simulink model "dynamic_vibration_absorb"  (R2020a)
settings: Solver=VariableStepAuto  StartTime=0.0  StopTime=50  RelTol=1e-3
PostLoadFcn:
  | m1=1/100
  | b=50
  | k1=50
  | m2=1/2
  | k2=0.9
settings Model: Creator=I3  LastModifiedBy=I3

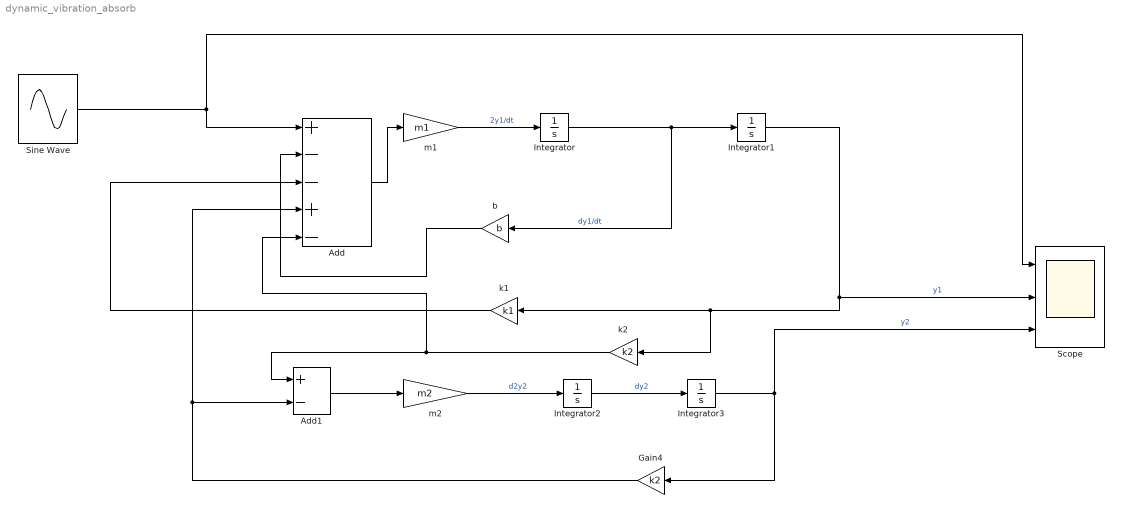
== system dynamic_vibration_absorb ==
  Add : Sum  Inputs=+--+-
  Add1 : Sum  Inputs=+-
  Gain4 : Gain  Gain=k2
  Integrator{,1..3} (4 alike) : Integrator
  Scope : Scope  NumInputPorts=3
  Sine Wave : Sin  Amplitude=2  Frequency=10  SampleTime=2*10^-4
  b : Gain  Gain=b
  k1 : Gain  Gain=k1
  k2 : Gain  Gain=k2
  m1 : Gain  Gain=m1
  m2 : Gain  Gain=m2
  wires:
  Integrator/1 -> b/1, Integrator1/1  "dy1/dt"
  Integrator1/1 -> k2/1, k1/1, Scope/2  "y1"
  Add/1 -> m1/1
  m1/1 -> Integrator/1  "2y1/dt"
  b/1 -> Add/2
  m2/1 -> Integrator2/1  "d2y2"
  Integrator2/1 -> Integrator3/1  "dy2"
  Integrator3/1 -> Scope/3, Gain4/1  "y2"
  Add1/1 -> m2/1
  k1/1 -> Add/3
  Gain4/1 -> Add/4, Add1/2
  k2/1 -> Add1/1, Add/5
  Sine Wave/1 -> Add/1, Scope/1
